simulink model "RST_Simulink"  (R2019b)
settings: Solver=VariableStepAuto  StartTime=0.0  StopTime=20  RelTol=1e-3
values from neighbouring files (symbols this model uses):
  Den = [1 -1.7 0.72]    [RST_Script.m]
  Num = [0 0.4 0.8]    [RST_Script.m]
  P = conv(Den,[1 -0.5])    [RST_Script.m]
  R = [0.4167 -0.7083 0.3000]    [RST_Script.m]
  S = conv([1 -1],[1 0.3333])    [RST_Script.m]
settings Model: Creator=PC  LastModifiedBy=PC

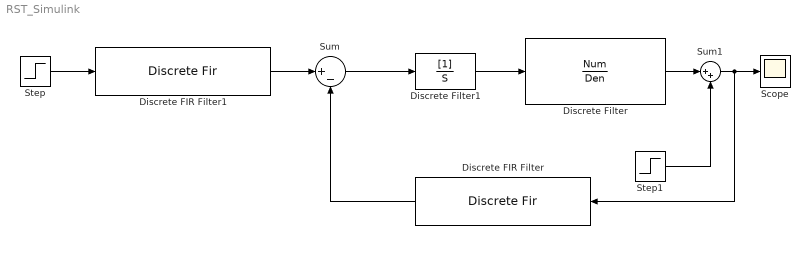
== system RST_Simulink ==
  Discrete FIR Filter : DiscreteFir  Coefficients=R
  Discrete FIR Filter1 : DiscreteFir  Coefficients=P/1.2
  Discrete Filter : DiscreteFilter  Numerator=Num  Denominator=Den
  Discrete Filter1 : DiscreteFilter  Denominator=S
  Scope : Scope
  Step : Step  Time=0  SampleTime=0
  Step1 : Step  Time=10  After=+0.5  SampleTime=0
  Sum : Sum  Inputs=|+-
  Sum1 : Sum  Inputs=|++
  wires:
  Discrete Filter1/1 -> Discrete Filter/1
  Discrete FIR Filter/1 -> Sum/2
  Sum/1 -> Discrete Filter1/1
  Discrete FIR Filter1/1 -> Sum/1
  Step/1 -> Discrete FIR Filter1/1
  Discrete Filter/1 -> Sum1/1
  Sum1/1 -> Discrete FIR Filter/1, Scope/1
  Step1/1 -> Sum1/2
